simulink model "quadcopter_model_discrete_z"  (R2019b)
settings: Solver=FixedStepAuto  StartTime=0.0  StopTime=5  RelTol=1e-3
undefined symbols (not defined in the file): DiscIntNeverNeededParam
libraries: simulink x3, simulink_extras x2
settings Model: Creator=edoardo  LastModifiedBy=edoardo
settings SFSimCC: CustomCodeUndefinedFunction=UseInterfaceOnly

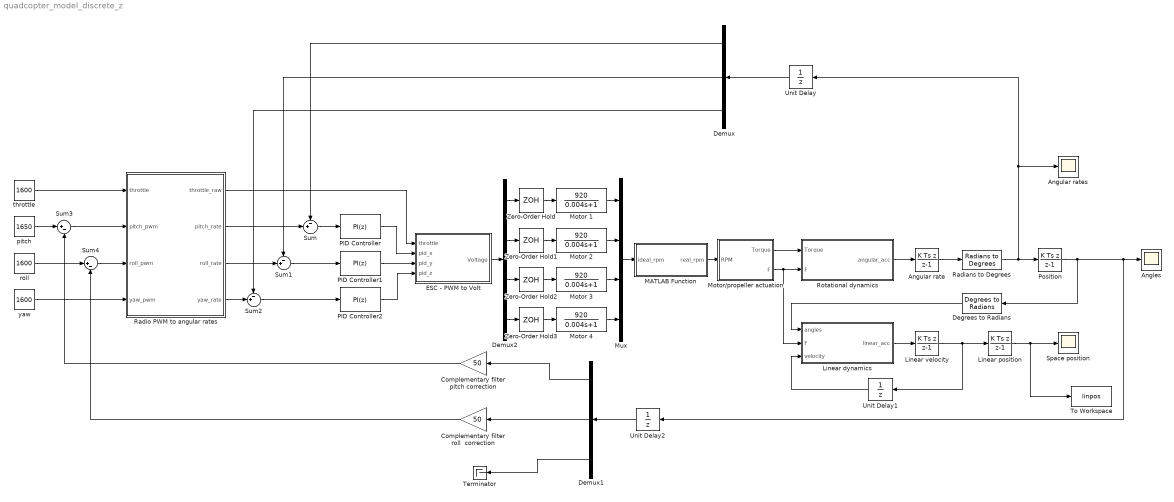
== system quadcopter_model_discrete_z ==
  "       Complementary filter pitch correction" : Gain  Gain=50
  "       Complementary filter roll  correction" : Gain  Gain=50
  "Angles " : Scope
  "Angular rate " : DiscreteIntegrator  IntegratorMethod=Integration: Backward Euler  SampleTime=-1  ICPrevOutput=DiscIntNeverNeededParam  ICPrevScaledInput=DiscIntNeverNeededParam
  Angular rates : Scope
  Degrees to Radians : simulink_extras/Transformations/Degrees to Radians
  Demux : Demux  Outputs=3
  Demux1 : Demux  Outputs=3
  Demux2 : Demux
  "ESC - PWM to Volt " : MATLAB Function  TreatAsAtomicUnit=on
  Linear position : DiscreteIntegrator  IntegratorMethod=Integration: Backward Euler  SampleTime=-1  ICPrevOutput=DiscIntNeverNeededParam  ICPrevScaledInput=DiscIntNeverNeededParam
  Linear velocity : DiscreteIntegrator  IntegratorMethod=Integration: Backward Euler  SampleTime=-1  ICPrevOutput=DiscIntNeverNeededParam  ICPrevScaledInput=DiscIntNeverNeededParam
  Linear dynamics : MATLAB Function  TreatAsAtomicUnit=on
  MATLAB Function : MATLAB Function  TreatAsAtomicUnit=on
  Motor {1..4} (4 alike) : TransferFcn  Numerator=[920]  Denominator=[0.004 1]
  Motor/propeller actuation : MATLAB Function  TreatAsAtomicUnit=on
  Mux : Mux
  PID Controller : simulink/Continuous/PID Controller  Controller=PI  Form=Parallel  TimeDomain=Discrete-time  SampleTime=0.004  IntegratorMethod=Backward Euler  FilterMethod=Backward Euler  ControllerParametersSource=internal  P=1.1  I=0.002  D=0.002  UseFilter=off  N=100  TunerSelectOption=Transfer Function Based (PID Tuner App)  InitialConditionSource=internal  InitialConditionForIntegrator=0  InitialConditionForFilter=0  DifferentiatorICPrevScaledInput=0  ExternalReset=none  TrackingMode=off  Kt=1  LimitOutput=on  UpperSaturationLimit=400  LowerSaturationLimit=-400  LinearizeAsGain=off  AntiWindupMode=clamping  Kb=1  POutMin=[]  POutMax=[]  IOutMin=[]  IOutMax=[]  DOutMin=[]  DOutMax=[]  NOutMin=[]  NOutMax=[]  SumOutMin=[]  SumOutMax=[]  SaturationOutMin=[]  SaturationOutMax=[]  PParamMin=[]  PParamMax=[]  IParamMin=[]  IParamMax=[]  DParamMin=[]  DParamMax=[]  NParamMin=[]  NParamMax=[]  KbParamMin=[]  KbParamMax=[]  KtParamMin=[]  KtParamMax=[]  KbOutMin=[]  KbOutMax=[]  KtOutMin=[]  KtOutMax=[]  IntegratorOutMin=[]  IntegratorOutMax=[]  FilterOutMin=[]  FilterOutMax=[]  SumI1OutMin=[]  SumI1OutMax=[]  SumI2OutMin=[]  SumI2OutMax=[]  SumI3OutMin=[]  SumI3OutMax=[]  SumI4OutMin=[]  SumI4OutMax=[]  SumDOutMin=[]  SumDOutMax=[]  DifferentiatorOutMin=[]  DifferentiatorOutMax=[]  FilterDiffOutCoefMin=[]  FilterDiffOutCoefMax=[]  ReciprocalOutMin=[]  ReciprocalOutMax=[]  SumDenOutMin=[]  SumDenOutMax=[]  SumNumOutMin=[]  SumNumOutMax=[]  DivideOutMin=[]  DivideOutMax=[]  IntegratorContinuousStateAttributes=''  IntegratorStateMustResolveToSignalObject=off  IntegratorRTWStateStorageClass=Auto  FilterContinuousStateAttributes=''  FilterStateMustResolveToSignalObject=off  FilterRTWStateStorageClass=Auto  ParallelPVariant=InternalParameters  IdealPVariant=Disabled  IVariant=InternalParameters  DVariant=Disabled  IntegratorVariant=Discrete  SatVariant=Enabled  AWVariant=DiscClampingParallel  PCopyVariant=Disabled  TRVariant=Disabled  FdbkBlocksVariant=Feedback  IdealPFdbkVariant=Passthrough  SatFdbkVariant=Passthrough  DerivativeFilterVariant=Disabled  NVariant=Disabled  NCopyVariant=Disabled_SignalSpec  FilterICVariant=Disabled  IntegratorICVariant=InternalICs  ExternalResetVariant=Disabled  TRSumVariant=Passthrough  SumFdbkVariant=Enabled  SumVariant=Sum_PI
  PID Controller1 : simulink/Continuous/PID Controller  Controller=PI  Form=Parallel  TimeDomain=Discrete-time  SampleTime=0.004  IntegratorMethod=Backward Euler  FilterMethod=Backward Euler  ControllerParametersSource=internal  P=1.1  I=0.002  D=0.005  UseFilter=off  N=37.6645512562197  TunerSelectOption=Transfer Function Based (PID Tuner App)  InitialConditionSource=internal  InitialConditionForIntegrator=0  InitialConditionForFilter=0  DifferentiatorICPrevScaledInput=0  ExternalReset=none  TrackingMode=off  Kt=1  LimitOutput=on  UpperSaturationLimit=400  LowerSaturationLimit=-400  LinearizeAsGain=off  AntiWindupMode=clamping  Kb=1  POutMin=[]  POutMax=[]  IOutMin=[]  IOutMax=[]  DOutMin=[]  DOutMax=[]  NOutMin=[]  NOutMax=[]  SumOutMin=[]  SumOutMax=[]  SaturationOutMin=[]  SaturationOutMax=[]  PParamMin=[]  PParamMax=[]  IParamMin=[]  IParamMax=[]  DParamMin=[]  DParamMax=[]  NParamMin=[]  NParamMax=[]  KbParamMin=[]  KbParamMax=[]  KtParamMin=[]  KtParamMax=[]  KbOutMin=[]  KbOutMax=[]  KtOutMin=[]  KtOutMax=[]  IntegratorOutMin=[]  IntegratorOutMax=[]  FilterOutMin=[]  FilterOutMax=[]  SumI1OutMin=[]  SumI1OutMax=[]  SumI2OutMin=[]  SumI2OutMax=[]  SumI3OutMin=[]  SumI3OutMax=[]  SumI4OutMin=[]  SumI4OutMax=[]  SumDOutMin=[]  SumDOutMax=[]  DifferentiatorOutMin=[]  DifferentiatorOutMax=[]  FilterDiffOutCoefMin=[]  FilterDiffOutCoefMax=[]  ReciprocalOutMin=[]  ReciprocalOutMax=[]  SumDenOutMin=[]  SumDenOutMax=[]  SumNumOutMin=[]  SumNumOutMax=[]  DivideOutMin=[]  DivideOutMax=[]  IntegratorContinuousStateAttributes=''  IntegratorStateMustResolveToSignalObject=off  IntegratorRTWStateStorageClass=Auto  FilterContinuousStateAttributes=''  FilterStateMustResolveToSignalObject=off  FilterRTWStateStorageClass=Auto  ParallelPVariant=InternalParameters  IdealPVariant=Disabled  IVariant=InternalParameters  DVariant=Disabled  IntegratorVariant=Discrete  SatVariant=Enabled  AWVariant=DiscClampingParallel  PCopyVariant=Disabled  TRVariant=Disabled  FdbkBlocksVariant=Feedback  IdealPFdbkVariant=Passthrough  SatFdbkVariant=Passthrough  DerivativeFilterVariant=Disabled  NVariant=Disabled  NCopyVariant=Disabled_SignalSpec  FilterICVariant=Disabled  IntegratorICVariant=InternalICs  ExternalResetVariant=Disabled  TRSumVariant=Passthrough  SumFdbkVariant=Enabled  SumVariant=Sum_PI
  PID Controller2 : simulink/Continuous/PID Controller  Controller=PI  Form=Parallel  TimeDomain=Discrete-time  SampleTime=0.004  IntegratorMethod=Backward Euler  FilterMethod=Backward Euler  ControllerParametersSource=internal  P=4  I=0.02  D=0.003  UseFilter=off  N=100  TunerSelectOption=Transfer Function Based (PID Tuner App)  InitialConditionSource=internal  InitialConditionForIntegrator=0  InitialConditionForFilter=0  DifferentiatorICPrevScaledInput=0  ExternalReset=none  TrackingMode=off  Kt=1  LimitOutput=on  UpperSaturationLimit=400  LowerSaturationLimit=-400  LinearizeAsGain=off  AntiWindupMode=clamping  Kb=1  POutMin=[]  POutMax=[]  IOutMin=[]  IOutMax=[]  DOutMin=[]  DOutMax=[]  NOutMin=[]  NOutMax=[]  SumOutMin=[]  SumOutMax=[]  SaturationOutMin=[]  SaturationOutMax=[]  PParamMin=[]  PParamMax=[]  IParamMin=[]  IParamMax=[]  DParamMin=[]  DParamMax=[]  NParamMin=[]  NParamMax=[]  KbParamMin=[]  KbParamMax=[]  KtParamMin=[]  KtParamMax=[]  KbOutMin=[]  KbOutMax=[]  KtOutMin=[]  KtOutMax=[]  IntegratorOutMin=[]  IntegratorOutMax=[]  FilterOutMin=[]  FilterOutMax=[]  SumI1OutMin=[]  SumI1OutMax=[]  SumI2OutMin=[]  SumI2OutMax=[]  SumI3OutMin=[]  SumI3OutMax=[]  SumI4OutMin=[]  SumI4OutMax=[]  SumDOutMin=[]  SumDOutMax=[]  DifferentiatorOutMin=[]  DifferentiatorOutMax=[]  FilterDiffOutCoefMin=[]  FilterDiffOutCoefMax=[]  ReciprocalOutMin=[]  ReciprocalOutMax=[]  SumDenOutMin=[]  SumDenOutMax=[]  SumNumOutMin=[]  SumNumOutMax=[]  DivideOutMin=[]  DivideOutMax=[]  IntegratorContinuousStateAttributes=''  IntegratorStateMustResolveToSignalObject=off  IntegratorRTWStateStorageClass=Auto  FilterContinuousStateAttributes=''  FilterStateMustResolveToSignalObject=off  FilterRTWStateStorageClass=Auto  ParallelPVariant=InternalParameters  IdealPVariant=Disabled  IVariant=InternalParameters  DVariant=Disabled  IntegratorVariant=Discrete  SatVariant=Enabled  AWVariant=DiscClampingParallel  PCopyVariant=Disabled  TRVariant=Disabled  FdbkBlocksVariant=Feedback  IdealPFdbkVariant=Passthrough  SatFdbkVariant=Passthrough  DerivativeFilterVariant=Disabled  NVariant=Disabled  NCopyVariant=Disabled_SignalSpec  FilterICVariant=Disabled  IntegratorICVariant=InternalICs  ExternalResetVariant=Disabled  TRSumVariant=Passthrough  SumFdbkVariant=Enabled  SumVariant=Sum_PI
  Position : DiscreteIntegrator  IntegratorMethod=Integration: Backward Euler  SampleTime=-1  ICPrevOutput=DiscIntNeverNeededParam  ICPrevScaledInput=DiscIntNeverNeededParam
  Radians to Degrees : simulink_extras/Transformations/Radians to Degrees
  Radio PWM to angular rates : MATLAB Function  TreatAsAtomicUnit=on
  "Rotational dynamics " : MATLAB Function  TreatAsAtomicUnit=on
  Space position : Scope
  Sum : Sum  Inputs=-+|
  Sum1 : Sum  Inputs=-+|
  Sum2 : Sum  Inputs=-+|
  Sum3 : Sum  Inputs=|+-
  Sum4 : Sum  Inputs=|+-
  Terminator : Terminator
  To Workspace : ToWorkspace  VariableName=linpos  SampleTime=-1
      settings: Save2DSignal=2-D array (concatenate along first dimension)
  Unit Delay : UnitDelay  SampleTime=-1  HasFrameUpgradeWarning=on
  Unit Delay1 : UnitDelay  SampleTime=-1  HasFrameUpgradeWarning=on
  Unit Delay2 : UnitDelay  SampleTime=-1  HasFrameUpgradeWarning=on
  Zero-Order Hold{,1..3} (4 alike) : ZeroOrderHold  SampleTime=-1
  pitch : Constant  Value=1650
  roll : Constant  Value=1600
  throttle : Constant  Value=1600
  yaw : Constant  Value=1600
  wires:
  Sum/1 -> PID Controller/1
  Sum1/1 -> PID Controller1/1
  Sum2/1 -> PID Controller2/1
  PID Controller/1 -> "ESC - PWM to Volt "/2(pid_x)
  PID Controller2/1 -> "ESC - PWM to Volt "/4(pid_z)
  PID Controller1/1 -> "ESC - PWM to Volt "/3(pid_y)
  "Rotational dynamics "/1(angular_acc) -> "Angular rate "/1
  "Angular rate "/1 -> Radians to Degrees/1
  throttle/1 -> Radio PWM to angular rates/1(throttle)
  Radio PWM to angular rates/1(throttle_raw) -> "ESC - PWM to Volt "/1(throttle)
  Radio PWM to angular rates/2(pitch_rate) -> Sum/2
  Radio PWM to angular rates/3(roll_rate) -> Sum1/2
  yaw/1 -> Radio PWM to angular rates/4(yaw_pwm)
  Radio PWM to angular rates/4(yaw_rate) -> Sum2/2
  Unit Delay/1 -> Demux/1
  Position/1 -> Degrees to Radians/1, "Angles "/1, Unit Delay2/1
  Demux1/2 -> "       Complementary filter roll  correction"/1
  Demux1/1 -> "       Complementary filter pitch correction"/1
  "       Complementary filter pitch correction"/1 -> Sum3/2
  "       Complementary filter roll  correction"/1 -> Sum4/2
  roll/1 -> Sum4/1
  pitch/1 -> Sum3/1
  Sum3/1 -> Radio PWM to angular rates/2(pitch_pwm)
  Sum4/1 -> Radio PWM to angular rates/3(roll_pwm)
  Demux1/3 -> Terminator/1
  Linear dynamics/1(linear_acc) -> Linear velocity/1
  Linear position/1 -> To Workspace/1, Space position/1
  Linear velocity/1 -> Linear position/1, Unit Delay1/1
  Degrees to Radians/1 -> Linear dynamics/1(angles)
  Unit Delay2/1 -> Demux1/1
  Unit Delay1/1 -> Linear dynamics/3(velocity)
  Demux/1 -> Sum/1
  Demux/2 -> Sum1/1
  Demux/3 -> Sum2/1
  Motor/propeller actuation/2(F) -> Linear dynamics/2(F), "Rotational dynamics "/2(F)
  Motor/propeller actuation/1(Torque) -> "Rotational dynamics "/1(Torque)
  Zero-Order Hold/1 -> Motor 1/1
  "ESC - PWM to Volt "/1(Voltage) -> Demux2/1
  Zero-Order Hold1/1 -> Motor 2/1
  Zero-Order Hold2/1 -> Motor 3/1
  Zero-Order Hold3/1 -> Motor 4/1
  Motor 1/1 -> Mux/1
  Motor 2/1 -> Mux/2
  Motor 3/1 -> Mux/3
  Motor 4/1 -> Mux/4
  Demux2/1 -> Zero-Order Hold/1
  Demux2/2 -> Zero-Order Hold1/1
  Demux2/3 -> Zero-Order Hold2/1
  Demux2/4 -> Zero-Order Hold3/1
  Mux/1 -> MATLAB Function/1(ideal_rpm)
  MATLAB Function/1(real_rpm) -> Motor/propeller actuation/1(RPM)
  Radians to Degrees/1 -> Position/1, Unit Delay/1, Angular rates/1

== matlab function quadcopter_model_discrete_z/Rotational dynamics  ==
  data: Torque input; angular_acc output; F input
function angular_acc = fcn(Torque, F)

    Moment      = [0 0 0];
    angular_acc = [0 0 0];
    Inertia     = [0.00305 0.00305 0.00611]; %Inertia for X,Y,Z
    axis_to_com = 0.1167;                    %distance between rotation axis and the center of mass of the vehicle

    
    Moment(1) = (F(2)+F(4))*axis_to_com-(F(1)+F(3))*axis_to_com;
    Moment(2) = (F(3)+F(4))*axis_to_com-(F(1)+F(2))*axis_to_com;
    Moment(3) = -Torque(1)+Torque(2)+Torque(3)-Torque(4);
        
    for i = 1:3
        angular_acc(i) = Moment(i)/Inertia(i);
    end

end

== matlab function quadcopter_model_discrete_z/ESC - PWM to Volt  ==
  data: throttle input; pid_x input; Voltage output; pid_y input; pid_z input

function Voltage = fcn(throttle,pid_x,pid_y,pid_z)
    %Parameters names, except the phisical ones, are directly taken from the C code implementation i.o.t. have 1:1 match  
    Voltage        = [0;0;0;0];
    
    if( throttle > 1800 )
        throttle = 1800;  %leave room for PID controller
    end
    
    Voltage(1) = throttle-pid_y-pid_x-pid_z;  %rear  right motor PWM
    Voltage(2) = throttle-pid_y+pid_x+pid_z;  %front right motor PWM
    Voltage(3) = throttle+pid_y-pid_x+pid_z;  %rear   left motor PWM
	Voltage(4) = throttle+pid_y+pid_x-pid_z;  %front  left motor PWM
   
    
    for i = 1:4  
        if( Voltage(i) > 2000 )
            Voltage(i) = 2000;
        end
        
        if( Voltage(i) < 1100 )
            Voltage(i) = 1100;
        end
        
        Voltage(i) = (Voltage(i)-1000)*0.0111;
    end

end

== matlab function quadcopter_model_discrete_z/Radio PWM to angular rates ==
  data: throttle input; throttle_raw output; pitch_pwm input; roll_pwm input; yaw_pwm input; pitch_rate output; roll_rate output; yaw_rate output
function [throttle_raw,pitch_rate,roll_rate,yaw_rate] = fcn(throttle,pitch_pwm,roll_pwm,yaw_pwm)

DEADBAND_UPPER_BOUND      = 1508;
DEADBAND_LOWER_BOUND      = 1492;
SETPOINT_PITCH_SPEED_RATE = 3.0;
SETPOINT_ROLL_SPEED_RATE  = 3.0;
SETPOINT_YAW_SPEED_RATE   = 3.0;

pitch_rate   = 0;
roll_rate    = 0;
yaw_rate     = 0;
throttle_raw = throttle;

if( pitch_pwm > DEADBAND_UPPER_BOUND )
    pitch_rate = ( pitch_pwm - DEADBAND_UPPER_BOUND ) / SETPOINT_PITCH_SPEED_RATE;
end
if( pitch_pwm < DEADBAND_LOWER_BOUND )
    pitch_rate = ( pitch_pwm - DEADBAND_LOWER_BOUND ) / SETPOINT_PITCH_SPEED_RATE;
end

if( roll_pwm > DEADBAND_UPPER_BOUND )
    roll_rate = ( roll_pwm - DEADBAND_UPPER_BOUND ) / SETPOINT_ROLL_SPEED_RATE;
end
if( roll_pwm < DEADBAND_LOWER_BOUND )
    roll_rate = ( roll_pwm - DEADBAND_LOWER_BOUND ) / SETPOINT_ROLL_SPEED_RATE;
end

if( yaw_pwm > DEADBAND_UPPER_BOUND )
    yaw_rate = ( yaw_pwm - DEADBAND_UPPER_BOUND ) / SETPOINT_YAW_SPEED_RATE;
end
if( yaw_pwm < DEADBAND_LOWER_BOUND )
    yaw_rate = ( yaw_pwm - DEADBAND_LOWER_BOUND ) / SETPOINT_YAW_SPEED_RATE;
end

end

== matlab function quadcopter_model_discrete_z/Linear dynamics ==
  data: angles input; F input; linear_acc output; velocity input
function linear_acc = fcn(angles,F,velocity)
    m   = 0.673;
    g   = 9.81;
    
    linear_acc = [0 0 0];
    Fprop      = [0 0 0];
    
    %Vettori di spinta (thrust vectors) vengono decomposti sulle componenti pitch e roll
    Fprop(1) = sin(angles(2)) * cos(angles(1)) * (F(1)+F(2)+F(3)+F(4));
    Fprop(2) = sin(angles(1)) * cos(angles(2)) * (F(1)+F(2)+F(3)+F(4));
    Fprop(3) = (F(1)+F(2)+F(3)+F(4)) * cos(angles(1)) * cos(angles(2));
    
    %Per lo yaw (asse Z) proietto l'angolo sul piano XY e trasformo le coordinate in un piano 2D
    ThetaXY  = atan2(Fprop(1), Fprop(2));
    XY2D     = sqrt(Fprop(1)^2 + Fprop(2)^2);

    %controllo la forza su Z per vedere se applicare ThetaXY a un angolo positivo o negativo 
    if( Fprop(3) >=0 )
        Fprop(1) = XY2D * cos(angles(3) + ThetaXY);
        Fprop(2) = XY2D * sin(angles(3) + ThetaXY);
    else
        Fprop(2) = XY2D * sin(-angles(3) + ThetaXY);
        Fprop(1) = XY2D * cos(-angles(3) + ThetaXY);
    end

    %su Z agisce anche in contrasto (o in favore) la forza peso del veicolo
    Fprop(3) = Fprop(3) - m * g;
    
    %calcolo le forze e trovo l'accelerazione lineare come formula inversa della seconda legge di Newton F = ma --> a = F/m
    for i = 1:3  
        linear_acc(i) = Fprop(i) / m;
    end
end

== matlab function quadcopter_model_discrete_z/Motor//propeller actuation ==
  data: RPM input; Torque output; F output
function [Torque, F] = fcn(RPM)
    
    Torque         = [0 0 0 0];
    F              = [0 0 0 0];

    for i = 1:4
        %RPM(i)     = -1.87*Voltage(i)^3-1.08*10^-14*Voltage(i)^2+920*Voltage(i)-3.79*10^-14;
        Ct         = 6.3*10^-19*RPM(i)^4-1.51*10^-14*RPM(i)^3+1.21*10^-10*RPM(i)^2-2.58*10^-7*RPM(i)+0.12;
        F(i)       = Ct*1.225*(RPM(i)/60)^2*0.001704;
        Torque(i)  = -1.79*10^-26*RPM(i)^6+4.63*10^-21*RPM(i)^5-1.37*10^-16*RPM(i)^4+1.5*10^-12*RPM(i)^3-5.96*10^-9*RPM(i)^2+1.11*10^-5*RPM(i)+4.52*10^-4;     
    end


end

== matlab function quadcopter_model_discrete_z/MATLAB Function ==
  data: ideal_rpm input; real_rpm output
function real_rpm = fcn(ideal_rpm)

    real_rpm = [0 0 0 0];
    
    for i = 1:4
        real_rpm(i) = -2.4*10^-9*ideal_rpm(i)^3-9.22*10^-21*ideal_rpm(i)^2+ideal_rpm(i)+9.36*10^-15;
    end

end
